simulink model "slave_model"  (R2020a)
settings: Solver=FixedStepDiscrete  StartTime=0.0  StopTime=1000.0  RelTol=1e-3  EnableMultiTasking=on
settings Model: SILPILModeSetting=veronly  ExtModeTrigDuration=2  Creator=davood  LastModifiedBy=davood
settings OptimizationCC: EnhancedBackFolding=on  PassReuseOutputArgsAs=Individual arguments  ZeroExternalMemoryAtStartup=off  ZeroInternalMemoryAtStartup=off  MaxStackSize=64  OptimizeBlockOrder=speed  DifferentSizesBufferReuse=on  OptimizationCustomize=off  EfficientTunableParamExpr=on
settings DebuggingCC: ParameterTunabilityLossMsg=error
settings HardwareCC: ProdBitPerInt=16  ProdBitPerPointer=16  ProdBitPerSizeT=16  ProdBitPerPtrDiffT=16  ProdLargestAtomicFloat=None  ProdWordSize=8  ProdHWDeviceType=Atmel->AVR
settings SFSimCC: MATLABDynamicMemAlloc=off
settings RTWCC: SystemTargetFile=ert.tlc  HardwareBoard=Arduino Uno  TLCOptions=-aInlineSetEventsForThisBaseRateFcn=TLC_FALSE -aSuppressMultiTaskScheduler=TLC_FALSE -aRateBasedStepFcn=1  TemplateMakefile=ert_default_tmf  GenerateReport=on  Toolchain=Arduino AVR  BuildConfiguration=Faster Runs  LaunchReport=on
settings CodeAppCC: ForceParamTrailComments=on  IgnoreCustomStorageClasses=off  OperatorAnnotations=on  SimulinkDataObjDesc=on  SFDataObjDesc=on  InsertBlockDesc=on
settings ERTTargetCC: SupportContinuousTime=on  SupportVariableSizeSignals=on  ExtModeStaticAllocSize=250

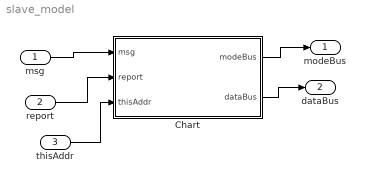
== system slave_model ==
  msg : Inport
  report : Inport  Port=2
  thisAddr : Inport  Port=3
  Chart : Stateflow chart  TreatAsAtomicUnit=on
  modeBus : Outport
  dataBus : Outport  Port=2
  wires:
  Chart/1(modeBus) -> modeBus/1
  Chart/2(dataBus) -> dataBus/1
  msg/1 -> Chart/1(msg)
  report/1 -> Chart/2(report)
  thisAddr/1 -> Chart/3(thisAddr)

== stateflow chart slave_model/Chart ==
  state init
  state addrValidation
  state sendReport
  state getMsg
  addrValidation -> sendReport [order 2] : [msg==thisAddr]{modeBus=0,dataBus=report}
  init -> addrValidation : [msg==1]
  (default) -> init
  sendReport -> getMsg : {modeBus=1}
  getMsg -> init [order 2] : [msg==0]
  addrValidation -> init [order 1] : [msg~=thisAddr]
  getMsg -> sendReport [order 1] : [msg~=0]{modeBus=0; dataBus=report}
  data: msg input uint8; modeBus output uint8; dataBus output uint8; report input uint8; thisAddr input uint8
